simulink model "thirdmodel"  (R2025a)
settings: Solver=daessc  StartTime=0.0  StopTime=1  RelTol=1e-3
libraries: spsRMSLib x3, spsACVoltageSourceLib x2, spsCurrentMeasurementLib x2, spsIdealSwitchLib x2, spsGroundLib x1, eeGeneralControl x1, spsMeanLib x1, spsParallelRLCLoadLib x1, spsSeriesRLCBranchLib x1, sps_lib x1, spsVariableResistorLib x1, spsVoltageMeasurementLib x1
settings Model: Creator=DELL  LastModifiedBy=DELL

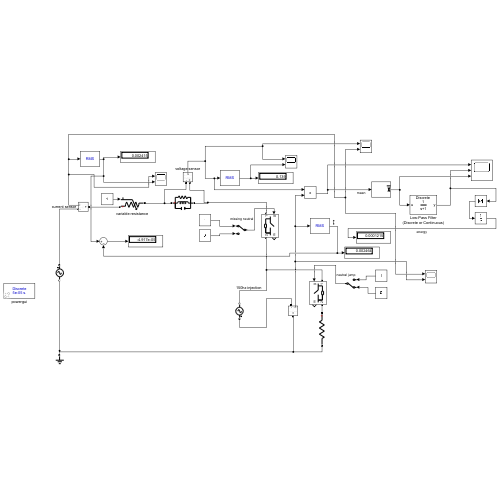
[thumbnail: Simulink's stored preview of the top-level diagram]
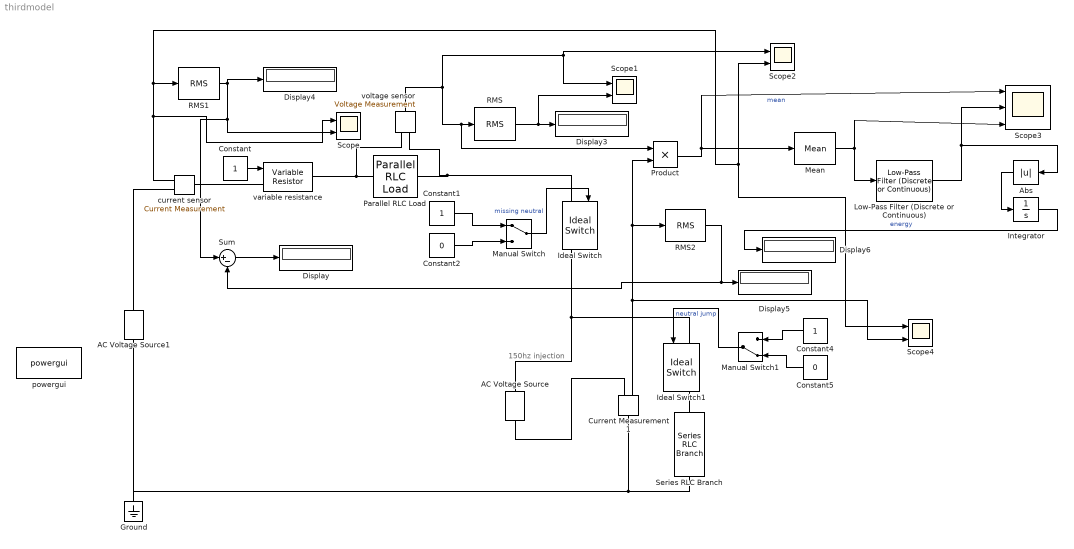
== system thirdmodel ==
  note: 150hz injection
  AC Voltage Source : spsACVoltageSourceLib/AC Voltage Source  Amplitude=40  Phase=0  Frequency=150  SampleTime=0  Measurements=None  BusType=swing  Pref=10e3  Qref=0  Qmin=-inf  Qmax=+inf
  AC Voltage Source1 : spsACVoltageSourceLib/AC Voltage Source  Amplitude=240*1.414  Phase=0  Frequency=50  SampleTime=0  Measurements=Voltage  BusType=swing  Pref=10e3  Qref=0  Qmin=-inf  Qmax=+inf
  Abs : Abs  SaturateOnIntegerOverflow=off
  Constant : Constant
  Constant1 : Constant
  Constant2 : Constant  Value=0
  Constant4 : Constant
  Constant5 : Constant  Value=0
  Current Measurement1 : spsCurrentMeasurementLib/Current Measurement  PhasorSimulation=off  OutputType=Complex  PSBequivalent=0
  Display{,3..6} (5 alike) : Display
  Ground : spsGroundLib/Ground  LConnTagsString=a
  Ideal Switch : spsIdealSwitchLib/Ideal Switch  Ron=0.001  Lon=0  IC=0  Rs=1e5  Cs=inf  Measurements=on
  Ideal Switch1 : spsIdealSwitchLib/Ideal Switch  Ron=0.00001  Lon=0  IC=0  Rs=1e5  Cs=inf  Measurements=on
  Integrator : Integrator
  Low-Pass Filter (Discrete or Continuous) : eeGeneralControl/Low-Pass Filter (Discrete or Continuous)  K=1  T=1  B=inf  A=-inf  init_option=Inherited from block input  x0=0  Ts=-1
  Manual Switch : ManualSwitch
  Manual Switch1 : ManualSwitch  CurrentSetting=0
  Mean : spsMeanLib/Mean  Freq=60  Vinit=0  Ts=0
  Parallel RLC Load : spsParallelRLCLoadLib/Parallel RLC Load  LConnTagsString=a  RConnTagsString=__new0  NominalVoltage=240  NominalFrequency=50  ActivePower=1000  InductivePower=100  CapacitivePower=100  Setx0=off  InitialVoltage=0  SetiL0=off  InitialCurrent=0  Measurements=None  LoadType=constant Z
      settings: AttributesFormatString=\n  LibrarySourceBlock=sps_lib/Passives/Parallel RLC Load
  Product : Product
  RMS : spsRMSLib/RMS  TrueRMS=on  Freq=50  RMSInit=120  Ts=0
  RMS1 : spsRMSLib/RMS  TrueRMS=on  Freq=50  RMSInit=120  Ts=0
  RMS2 : spsRMSLib/RMS  TrueRMS=on  Freq=50  RMSInit=120  Ts=0
  Scope{,1..2,4} (4 alike) : Scope  NumInputPorts=2
      Scope settings: ActiveDisplayYMinimum=-22.153677301376991  ActiveDisplayYMaximum=135.79485303348633
      Scope1 settings: ActiveDisplayYMinimum=-416.65401839919673  ActiveDisplayYMaximum=417.554375787498
      Scope2 settings: PlotAsMagnitudePhase=on  ActiveDisplayYMinimum=-62.378825783141679  ActiveDisplayYMaximum=376.17144070094577  DataLoggingVariableName=ScopeData2
      Scope4 settings: PlotAsMagnitudePhase=on  ActiveDisplayYMinimum=-0.69606419546097364  ActiveDisplayYMaximum=6.4990043729065166  DataLoggingVariableName=ScopeData4
  Scope3 : Scope  NumInputPorts=3
      settings: ActiveDisplayYMinimum=-223.92257300772079  ActiveDisplayYMaximum=1928.7058139870319  DataLoggingVariableName=ScopeData3
  Series RLC Branch : spsSeriesRLCBranchLib/Series RLC Branch  LConnTagsString=__new0  RConnTagsString=__new0  BranchType=R  Resistance=0.0001  Inductance=1e-3  SetiL0=off  InitialCurrent=0  Capacitance=1e-6  Setx0=off  InitialVoltage=0  Measurements=None
  Sum : Sum  Inputs=|+-
  current sensor : spsCurrentMeasurementLib/Current Measurement  PhasorSimulation=off  OutputType=Complex  PSBequivalent=0
  powergui : sps_lib/powergui  Priority=1  SimulationMode=Discrete  SampleTime=50e-6  frequency=60  Iterations=50  frequencyindice=50  Pbase=100e6  ErrMax=1e-4  UnitsV=kV  UnitsW=MW  buscounter=0  FunctionMessages=off  echomessages=off  EnableUseOfTLC=off  CurrentSourceSwitches=off  DisableSnubberDevices=off  DisableRonSwitches=off  DisableVfSwitches=off  DisplayEquations=off  AutomaticDiscreteSolvers=off  SolverType=Tustin/Backward Euler (TBE)  Interpol=off  ExternalGateDelay=off  methode=off  Ts=100  x0status=blocks  SPID=on  SwTol=0  HookPort=off  NonlinearTolerance=1e-4  nMaxIteration=100  ContinueOnMaxIteration=off  RestoreLinks=warning  ResistiveCurrentMeasurement=off  Frange=[0:2:500]  Ylog=off  Xlog=on  ShowGrid=off  save=off  variable=ZData  structure=0  ZoomFFT=off  StartTime=0.0  cycles=1  DisplayStyle=1  fundamental=60  FreqAxis=off  MaxFrequency=1000  frequencyindicesteady=1  RmsSteady=1  display=off
  variable resistance : spsVariableResistorLib/Variable Resistor  Rabsmin=1e-3
      settings: LibrarySourceBlock=sps_lib/Passives/Variable Resistor
  voltage sensor : spsVoltageMeasurementLib/Voltage Measurement  PhasorSimulation=off  OutputType=Complex  PSBequivalent=0
  wires:
  current sensor/1 -> Scope/1, RMS1/1, Scope4/1, Scope2/2
  Current Measurement1/1 -> Scope4/2, Product/2, RMS2/1
  voltage sensor/1 -> Product/1, RMS/1, Scope1/1, Scope2/1
  Constant/1 -> variable resistance/1
  RMS/1 -> Scope1/2, Display3/1
  RMS2/1 -> Sum/2, Display5/1
  RMS1/1 -> Sum/1, Scope/2, Display4/1
  Product/1 -> Scope3/1, Mean/1  "mean"
  Mean/1 -> Low-Pass Filter (Discrete or Continuous)/1, Scope3/3
  Abs/1 -> Integrator/1
  Integrator/1 -> Display6/1  "energy"
  Constant1/1 -> Manual Switch/1
  Constant2/1 -> Manual Switch/2
  Low-Pass Filter (Discrete or Continuous)/1 -> Scope3/2, Abs/1
  Manual Switch/1 -> Ideal Switch/1  "missing neutral"
  Constant5/1 -> Manual Switch1/2
  Manual Switch1/1 -> Ideal Switch1/1  "neutral jump"
  Constant4/1 -> Manual Switch1/1
  Sum/1 -> Display/1
  connections:
  Parallel RLC Load/RConn1 -- Ideal Switch/LConn1 -- voltage sensor/LConn1
  variable resistance/RConn1 -- voltage sensor/LConn2 -- Parallel RLC Load/LConn1
  current sensor/RConn1 -- AC Voltage Source1/RConn1
  current sensor/LConn1 -- variable resistance/LConn1
  Ideal Switch/RConn1 -- AC Voltage Source/LConn1 -- Ideal Switch1/LConn1
  Current Measurement1/LConn1 -- Ground/LConn1 -- AC Voltage Source1/LConn1 -- Series RLC Branch/RConn1
  Series RLC Branch/LConn1 -- Ideal Switch1/RConn1
  AC Voltage Source/RConn1 -- Current Measurement1/RConn1
